simulink model "line_diagram"  (R2026a)
settings: Solver=ode15s  StopTime=15.0
libraries: fl_lib x25, nesl_utility x7, ee_lib x6
settings Model: Creator=zoyab  LastModifiedBy=zoyab
settings SimscapeCC: SimscapeNominalValues="[{\"value\":\"1\",\"unit\":\"A\"},{\"value\":\"1\",\"unit\":\"bar\"},{\"value\":\"1\",\"unit\":\"cm^2\"},{\"value\":\"1\",\"unit\":\"cm^3/s\"},{\"value\":\"1\",\"unit\":\"kJ/kg\"},{\"value\":\"1\",\"unit\":\"kW\"},{\"value\":\"1\",\"unit\":\"l\"},{\"value\":\"1\",\"unit\":\"N\"},{\"value\":\"1\",\"unit\":\"N*m\"},{\"value\":\"1\",\"unit\":\"V\"}]"  SimscapeLogType=none  SimscapeLogDataHistory=5000.0

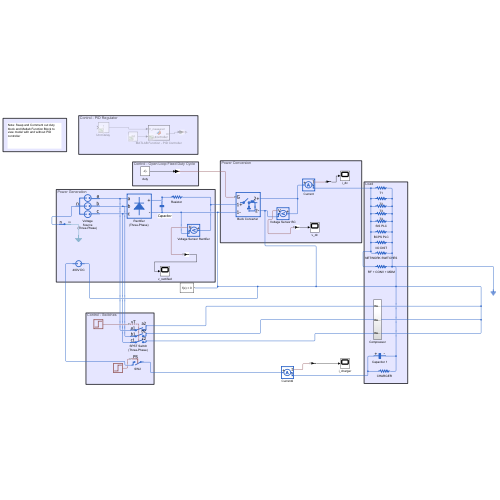
[thumbnail: Simulink's stored preview of the top-level diagram]
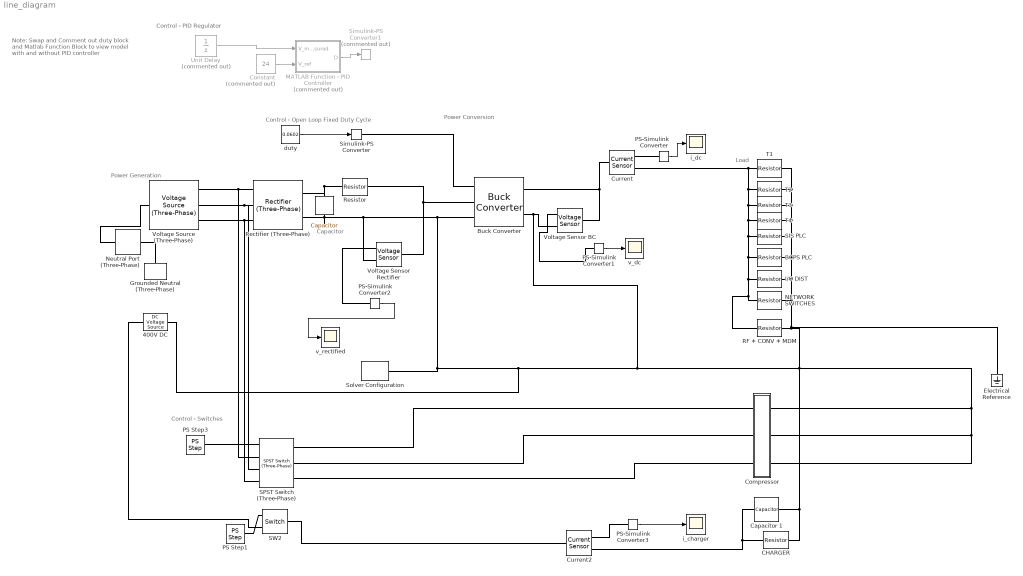
== system line_diagram ==
  note: Control - Open Loop Fixed Duty Cycle
  note: Note: Swap and Comment out duty block and Matlab Function Block to view model with and without PID controller
  note: Control - PID Regulator
  note: Control - Switches
  note: Load
  note: Power Conversion
  note: Power Generation
  note: Capacitor
  " " : fl_lib/Electrical/Electrical Elements/Capacitor  c=2200 uF  r=1e-6 Ohm  g=0 1/Ohm  i_specify=off  i_priority=None  i=0 A  i_nominal_specify=off  i_nominal_value=1  i_nominal_unit=A  v_specify=off  v_priority=None  v=409 V  v_nominal_specify=off  v_nominal_value=1  v_nominal_unit=V  vc_specify=off  vc_priority=High  vc=0 V  vc_nominal_specify=off  vc_nominal_value=1  vc_nominal_unit=V
  400V DC : fl_lib/Electrical/Electrical Sources/DC Voltage Source  v0=400 V
  BCPS PLC : fl_lib/Electrical/Electrical Elements/Resistor  R=30 Ohm  i_specify=off  i_priority=None  i=0 A  i_nominal_specify=off  i_nominal_value=1  i_nominal_unit=A  v_specify=off  v_priority=None  v=0 V  v_nominal_specify=off  v_nominal_value=1  v_nominal_unit=V
  "Buck Converter " : ee_lib/Semiconductors & Converters/Converters/Buck Converter  port_option=ee.enum.controlport.ps  device_type=ee.enum.converters.switchingdevice.averaged  Vf=0.8 V  Ron=0.001 Ohm  Rds=0.001 Ohm  Goff=1e-5 1/Ohm  Vgt=1 V  Vgt_off=-1 V  Ih=1 A  Vth=6 V  K=0  diode_param=ee.enum.converters.protectiondiode.nodynamics  diode_Vf=0.8 V  diode_Ron=0.001 Ohm  diode_Goff=1e-5 1/Ohm  diode_C=50 nF  diode_iRM=-235 A  diode_iF=300 A  diode_idot=-50 A/us  diode_trr_param=ee.enum.converters.diodetrr.trr_factor  diode_trr_factor=3  diode_trr=15 us  diode_Qrr=1500 s*uA  Lf=6.8e-6 H  Rl=1e-3 Ohm  Cf=47e-6 F  Rf=1e-6 Ohm  snubber_type=ee.enum.converters.snubber.exclude  Cs=1e-7 F  Rs=0.1 Ohm  iL_specify=off  iL_priority=High  iL=0 A  iL_nominal_specify=off  iL_nominal_value=1  iL_nominal_unit=A  vc_specify=off  vc_priority=High  vc=0 V  vc_nominal_specify=off  vc_nominal_value=1  vc_nominal_unit=V
  CHARGER : fl_lib/Electrical/Electrical Elements/Resistor  R=45.33 Ohm  i_specify=off  i_priority=None  i=0 A  i_nominal_specify=off  i_nominal_value=1  i_nominal_unit=A  v_specify=off  v_priority=None  v=0 V  v_nominal_specify=off  v_nominal_value=1  v_nominal_unit=V
  Capacitor 1 : fl_lib/Electrical/Electrical Elements/Capacitor  c=1 uF  r=1e-6 Ohm  g=0 1/Ohm  i_specify=off  i_priority=None  i=0 A  i_nominal_specify=off  i_nominal_value=1  i_nominal_unit=A  v_specify=off  v_priority=None  v=409 V  v_nominal_specify=off  v_nominal_value=1  v_nominal_unit=V  vc_specify=off  vc_priority=High  vc=0 V  vc_nominal_specify=off  vc_nominal_value=1  vc_nominal_unit=V
  Compressor : Subsystem
  Constant : Constant  Commented=on  Value=24
  Current : fl_lib/Electrical/Electrical Sensors/Current Sensor
  Current2 : fl_lib/Electrical/Electrical Sensors/Current Sensor
  Electrical Reference : fl_lib/Electrical/Electrical Elements/Electrical Reference
  Grounded Neutral (Three-Phase) : ee_lib/Connectors & References/Grounded Neutral (Three-Phase)  port_option=ee.enum.threePhasePort.composite
  I/O DIST : fl_lib/Electrical/Electrical Elements/Resistor  R=11.52 Ohm  i_specify=off  i_priority=None  i=0 A  i_nominal_specify=off  i_nominal_value=1  i_nominal_unit=A  v_specify=off  v_priority=None  v=0 V  v_nominal_specify=off  v_nominal_value=1  v_nominal_unit=V
  MATLAB Function - PID Controller : MATLAB Function  Commented=on  TreatAsAtomicUnit=on
  NETWORK SWITCHES : fl_lib/Electrical/Electrical Elements/Resistor  R=14.4 Ohm  i_specify=off  i_priority=None  i=0 A  i_nominal_specify=off  i_nominal_value=1  i_nominal_unit=A  v_specify=off  v_priority=None  v=0 V  v_nominal_specify=off  v_nominal_value=1  v_nominal_unit=V
  Neutral Port (Three-Phase) : ee_lib/Connectors & References/Neutral Port (Three-Phase)  port_option=ee.enum.threePhasePort.composite  G_parasitic=1e-12 1/Ohm
  PS Step1 : fl_lib/Physical Signals/Sources/PS Step  step_time=10 s  initial_value=0  final_value=1
  PS Step3 : fl_lib/Physical Signals/Sources/PS Step  step_time=5 s  initial_value=0  final_value=1
  PS-Simulink Converter{,1..3} (4 alike) : nesl_utility/PS-Simulink Converter  PhysicalDomain=network_engine_domain  SubClassName=ps_output  LeftPortType=input  RightPortType=output  PseudoPeriodic=off  Frequencies=[]  VectorFormat=inherit  Unit=inherit  AffineConversion=off
  RF + CONV + MDM : fl_lib/Electrical/Electrical Elements/Resistor  R=23.04 Ohm  i_specify=off  i_priority=None  i=0 A  i_nominal_specify=off  i_nominal_value=1  i_nominal_unit=A  v_specify=off  v_priority=None  v=0 V  v_nominal_specify=off  v_nominal_value=1  v_nominal_unit=V
  "Rectifier (Three-Phase) " : ee_lib/Semiconductors & Converters/Converters/Rectifier (Three-Phase)  port_option=ee.enum.threePhasePort.expanded  Vf=0.8 V  Ron=0.001 Ohm  Goff=1e-5 1/Ohm  model_dynamics=ee.enum.converters.diode.nodynamics  C=50 nF  iRM=-235 A  iF=300 A  idot=-50 A/us  trr_param=ee.enum.converters.diodetrr.trr_factor  trr_factor=3  trr=15 us  Qrr=1500 s*uA
  "Resistor " : fl_lib/Electrical/Electrical Elements/Resistor  R=5 Ohm  i_specify=off  i_priority=None  i=0 A  i_nominal_specify=off  i_nominal_value=1  i_nominal_unit=A  v_specify=off  v_priority=None  v=0 V  v_nominal_specify=off  v_nominal_value=1  v_nominal_unit=V
  SIS PLC : fl_lib/Electrical/Electrical Elements/Resistor  R=48 Ohm  i_specify=off  i_priority=None  i=0 A  i_nominal_specify=off  i_nominal_value=1  i_nominal_unit=A  v_specify=off  v_priority=None  v=0 V  v_nominal_specify=off  v_nominal_value=1  v_nominal_unit=V
  "SPST Switch (Three-Phase) " : ee_lib/Switches & Breakers/SPST Switch (Three-Phase)  port_option=ee.enum.threePhasePort.expanded  control_port_option=ee.enum.controlport.ps  R_closed=0.001 Ohm  G_open=1e-6 1/Ohm  threshold=0.5 V
  SW2 : fl_lib/Electrical/Electrical Elements/Switch  R_closed=0.01 Ohm  G_open=1e-8 1/Ohm  Threshold=0.5  i_specify=off  i_priority=None  i=0 A  i_nominal_specify=off  i_nominal_value=1  i_nominal_unit=A  v_specify=off  v_priority=None  v=0 V  v_nominal_specify=off  v_nominal_value=1  v_nominal_unit=V
  Simulink-PS Converter : nesl_utility/Simulink-PS Converter  PhysicalDomain=network_engine_domain  SubClassName=ps_input  LeftPortType=input  RightPortType=output  PseudoPeriodic=off  Frequencies=[]  NoiseDistribution=none  NoiseParameters=[]  Unit=1  AffineConversion=off  FilteringAndDerivatives=provide  SimscapeFilterOrder=1  InputFilterTimeConstant=0.001  UdotUserProvided=0
  Simulink-PS Converter1 : nesl_utility/Simulink-PS Converter  Commented=on  PhysicalDomain=network_engine_domain  SubClassName=ps_input  LeftPortType=input  RightPortType=output  PseudoPeriodic=off  Frequencies=[]  NoiseDistribution=none  NoiseParameters=[]  Unit=1  AffineConversion=off  FilteringAndDerivatives=provide  SimscapeFilterOrder=1  InputFilterTimeConstant=0.001  UdotUserProvided=0
  Solver Configuration : nesl_utility/Solver Configuration  PhysicalDomain=network_engine_domain  SubClassName=solver  LeftPortType=input  RightPortType=generic  Tones=[]  Harmonics=[]  SimulateNoise=off  Profile=off  UseLocalSampling=off  EnableSwitchedLinearOptims=on  FrequencyDomain=off  UseCCode=off  RelTol=0.001  AbsTol=0.001  MinStep=1e-09  ToWorkspace=off  RevertToSquareIcSolve=off  NumHomotopyIterations=100  PhasorMode=off  PhasorModeNumHarmonics=1  ConsistencySolver=NEWTON_XTOL_AFTER_FTOL  CanonicalOrdering=UNORDERED  OptimizeIntermediates=UNOPTIMIZED  IndexReductionMethod=DerivativeReplacement  DoDC=off  ResidualTolerance=1e-09  ConsistencyTolSource=GLOBAL  ConsistencyAbsTol=0.001  ConsistencyRelTol=0.001  ConsistencyTolFactor=0.001  UseLocalSolver=off  LocalSolverChoice=NE_BACKWARD_EULER_ADVANCER  ResolveIndetEquations=on  FunctionEvalNumThread=1  LocalSolverSampleTime=0.001  DoFixedCost=off  MaxNonlinIter=3  MaxModeIter=2  ComputeImpulses=off  ImpulseIterations=2  LinearAlgebra=auto  LinearAlgebraNumThread=0  EquationFormulation=NE_TIME_EF  DelaysMemoryBudget=1024  AutomaticFiltering=on  FilteringTimeConstant=0.001  PartitionStorageMethod=AS_NEEDED  PartitionMemoryBudget=1024  PartitionMethod=ROBUST  MultibodyUseLocalSolver=off  MultibodyLocalSolverChoice=ODE1  MultibodyLocalSolverSampleTime=0.001
  T1 : fl_lib/Electrical/Electrical Elements/Resistor  R=46.154 Ohm  i_specify=off  i_priority=None  i=0 A  i_nominal_specify=off  i_nominal_value=1  i_nominal_unit=A  v_specify=off  v_priority=None  v=0 V  v_nominal_specify=off  v_nominal_value=1  v_nominal_unit=V
  T2 : fl_lib/Electrical/Electrical Elements/Resistor  R=21.365 Ohm  i_specify=off  i_priority=None  i=0 A  i_nominal_specify=off  i_nominal_value=1  i_nominal_unit=A  v_specify=off  v_priority=None  v=0 V  v_nominal_specify=off  v_nominal_value=1  v_nominal_unit=V
  T3 : fl_lib/Electrical/Electrical Elements/Resistor  R=81.586 Ohm  i_specify=off  i_priority=None  i=0 A  i_nominal_specify=off  i_nominal_value=1  i_nominal_unit=A  v_specify=off  v_priority=None  v=0 V  v_nominal_specify=off  v_nominal_value=1  v_nominal_unit=V
  T4 : fl_lib/Electrical/Electrical Elements/Resistor  R=150 Ohm  i_specify=off  i_priority=None  i=0 A  i_nominal_specify=off  i_nominal_value=1  i_nominal_unit=A  v_specify=off  v_priority=None  v=0 V  v_nominal_specify=off  v_nominal_value=1  v_nominal_unit=V
  "Unit Delay " : UnitDelay  Commented=on  SampleTime=1e-4
  "Voltage Source (Three-Phase) " : ee_lib/Sources/Voltage Source (Three-Phase)  vline_rms=494 V  shift=0 deg  freq=50 Hz  impedance_option=0  SShortCircuit=1e9 A*V  XR=15  R=0.1 Ohm  L=1e-4 H  harmonic_option=0  harmonic_orders=[5, 7, 11, 13]  harmonic_ratios=[.1, .1, .1, .1]  G_parasitic=0 1/Ohm  I_specify=off  I_priority=None  I=[0, 0, 0] A  I_nominal_specify=off  I_nominal_value=1  I_nominal_unit=A
  Voltage Sensor BC : fl_lib/Electrical/Electrical Sensors/Voltage Sensor
  Voltage Sensor Rectifier : fl_lib/Electrical/Electrical Sensors/Voltage Sensor
  duty : Constant  Value=0.0602
  i_charger : Scope
      settings: ActiveDisplayYMinimum=8.8222293099130109  ActiveDisplayYMaximum=8.82223573292513  DataLoggingVariableName=ScopeData3
  i_dc : Scope
      settings: ActiveDisplayYMinimum=8.2085519745514386  ActiveDisplayYMaximum=8.215670150092679
  v_dc : Scope
      settings: ActiveDisplayYMinimum=16.260004980346551  ActiveDisplayYMaximum=36.554844425367804
  v_rectified : Scope
      settings: ActiveDisplayYMinimum=400.03129980668893  ActiveDisplayYMaximum=400.064175740174  DataLoggingVariableName=ScopeData2
  wires:
  PS-Simulink Converter2/1 -> v_rectified/1
  PS-Simulink Converter/1 -> i_dc/1
  duty/1 -> Simulink-PS Converter/1
  PS-Simulink Converter3/1 -> i_charger/1
  PS-Simulink Converter1/1 -> v_dc/1
  "Unit Delay "/1 -> MATLAB Function - PID Controller/1(V_measured)
  MATLAB Function - PID Controller/1(D) -> Simulink-PS Converter1/1
  Constant/1 -> MATLAB Function - PID Controller/2(V_ref)
  connections:
  "Rectifier (Three-Phase) "/RConn1 -- " "/LConn1 -- "Resistor "/LConn1
  T1/LConn1 -- Current/RConn2 -- NETWORK SWITCHES/LConn1 -- RF + CONV + MDM/LConn1 -- I/O DIST/LConn1 -- BCPS PLC/LConn1 -- SIS PLC/LConn1 -- T4/LConn1 -- T3/LConn1 -- T2/LConn1
  Voltage Sensor BC/LConn1 -- Current/LConn1 -- "Buck Converter "/RConn1
  Current/RConn1 -- PS-Simulink Converter/LConn1
  Voltage Sensor BC/RConn1 -- PS-Simulink Converter1/LConn1
  PS-Simulink Converter2/LConn1 -- Voltage Sensor Rectifier/RConn1
  Neutral Port (Three-Phase)/RConn1 -- "Voltage Source (Three-Phase) "/LConn1
  Neutral Port (Three-Phase)/LConn1 -- Grounded Neutral (Three-Phase)/LConn1
  CHARGER/LConn1 -- Capacitor 1/LConn1 -- Current2/RConn2
  "Buck Converter "/LConn2 -- Voltage Sensor Rectifier/LConn1 -- "Resistor "/RConn1
  PS Step1/RConn1 -- SW2/RConn1
  "Rectifier (Three-Phase) "/LConn3 -- "Voltage Source (Three-Phase) "/RConn3 -- "SPST Switch (Three-Phase) "/LConn4
  "Rectifier (Three-Phase) "/LConn2 -- "Voltage Source (Three-Phase) "/RConn2 -- "SPST Switch (Three-Phase) "/LConn3
  "Rectifier (Three-Phase) "/LConn1 -- "Voltage Source (Three-Phase) "/RConn1 -- "SPST Switch (Three-Phase) "/LConn2
  PS Step3/RConn1 -- "SPST Switch (Three-Phase) "/LConn1
  "SPST Switch (Three-Phase) "/RConn3 -- Compressor/LConn3
  "SPST Switch (Three-Phase) "/RConn1 -- Compressor/LConn1
  "SPST Switch (Three-Phase) "/RConn2 -- Compressor/LConn2
  Voltage Sensor BC/RConn2 -- T1/RConn1 -- T2/RConn1 -- T3/RConn1 -- T4/RConn1 -- SIS PLC/RConn1 -- BCPS PLC/RConn1 -- I/O DIST/RConn1 -- NETWORK SWITCHES/RConn1 -- Electrical Reference/LConn1 -- RF + CONV + MDM/RConn1 -- Compressor/RConn3 -- Compressor/RConn2 -- Compressor/RConn1 -- CHARGER/RConn1 -- Capacitor 1/RConn1 -- Solver Configuration/RConn1 -- "Buck Converter "/LConn3 -- "Rectifier (Three-Phase) "/RConn2 -- " "/RConn1 -- Voltage Sensor Rectifier/RConn2 -- 400V DC/RConn1 -- "Buck Converter "/RConn2
  Current2/RConn1 -- PS-Simulink Converter3/LConn1
  Current2/LConn1 -- SW2/LConn1
  SW2/RConn2 -- 400V DC/LConn1
  Simulink-PS Converter/RConn1 -- "Buck Converter "/LConn1

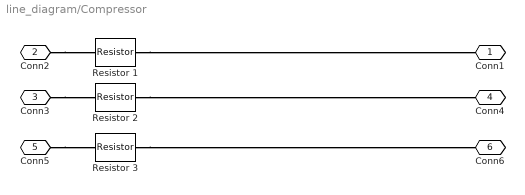
== system line_diagram/Compressor ==
  Resistor 1 : fl_lib/Electrical/Electrical Elements/Resistor  R=35.2 Ohm  i_specify=off  i_priority=None  i=0 A  i_nominal_specify=off  i_nominal_value=1  i_nominal_unit=A  v_specify=off  v_priority=None  v=0 V  v_nominal_specify=off  v_nominal_value=1  v_nominal_unit=V
  Resistor 2 : fl_lib/Electrical/Electrical Elements/Resistor  R=35.2 Ohm  i_specify=off  i_priority=None  i=0 A  i_nominal_specify=off  i_nominal_value=1  i_nominal_unit=A  v_specify=off  v_priority=None  v=0 V  v_nominal_specify=off  v_nominal_value=1  v_nominal_unit=V
  Resistor 3 : fl_lib/Electrical/Electrical Elements/Resistor  R=35.2 Ohm  i_specify=off  i_priority=None  i=0 A  i_nominal_specify=off  i_nominal_value=1  i_nominal_unit=A  v_specify=off  v_priority=None  v=0 V  v_nominal_specify=off  v_nominal_value=1  v_nominal_unit=V
  Conn1 : PMIOPort  Side=Right
  Conn2 : PMIOPort  Port=2  Side=Left
  Conn3 : PMIOPort  Port=3  Side=Left
  Conn4 : PMIOPort  Port=4  Side=Right
  Conn5 : PMIOPort  Port=5  Side=Left
  Conn6 : PMIOPort  Port=6  Side=Right
  connections:
  Resistor 2/RConn1 -- Conn4/RConn1
  Resistor 1/RConn1 -- Conn1/RConn1
  Conn5/RConn1 -- Resistor 3/LConn1
  Conn2/RConn1 -- Resistor 1/LConn1
  Resistor 3/RConn1 -- Conn6/RConn1
  Conn3/RConn1 -- Resistor 2/LConn1

== matlab function line_diagram/MATLAB Function - PID Controller ==
  data: V_measured input; D output; V_ref input
function D = pid_controller(V_measured, V_ref)
    persistent e_prev e_prev2 D_prev;
    if isempty(D_prev)
        e_prev  = 0;
        e_prev2 = 0;
        D_prev  = 0.050; 
    end
  
    Kp = 0.001;  
    Ki = 0.1;    
    Kd = 0.0;    
    Ts = 1e-4;
    
    e = V_ref - V_measured;
    
    delta_D = Kp * (e - e_prev) ...
            + Ki * Ts * e ...
            + (Kd / Ts) * (e - 2*e_prev + e_prev2);
    
    D = D_prev + delta_D;   
    D = max(0.005, min(0.95, D));
    
    e_prev2 = e_prev;
    e_prev  = e;
    D_prev  = D;
end
